simulink model "ex_bus_assignment_signal"  (R2019b)
settings: Solver=VariableStepAuto  StartTime=0.0  StopTime=10.0  RelTol=1e-3
settings Model: Creator=The MathWorks, Inc.  LastModifiedBy=bhisma
settings DebuggingCC: ArithmeticOperatorsInVariantConditions=warning
settings SFSimCC: SimUseLocalCustomCode=off  CustomCodeUndefinedFunction=UseInterfaceOnly
settings RTWCC: RTWUseLocalCustomCode=off
settings CodeAppCC: StateflowObjectComments=on
settings ConfigComp: CovMetricSettings=dswe

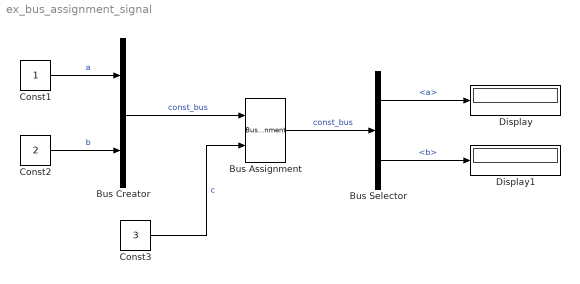
== system ex_bus_assignment_signal ==
  Bus Assignment : BusAssignment  AssignedSignals=a
  Bus Creator : BusCreator  Inputs=2
  Bus Selector : BusSelector  OutputSignals=a,b
  Const1 : Constant
  Const2 : Constant  Value=2
  Const3 : Constant  Value=3
  Display : Display
  Display1 : Display
  wires:
  Const1/1 -> Bus Creator/1  "a"
  Const2/1 -> Bus Creator/2  "b"
  Bus Creator/1 -> Bus Assignment/1  "const_bus"
  Const3/1 -> Bus Assignment/2  "c"
  Bus Assignment/1 -> Bus Selector/1  "const_bus"
  Bus Selector/1 -> Display/1  "<a>"
  Bus Selector/2 -> Display1/1  "<b>"
